simulink model "CN_filter"  (R2015b)
settings: Solver=VariableStepAuto  StartTime=0.0  StopTime=10.0  RelTol=1e-3
values from neighbouring files (symbols this model uses):
  FS = 0.2    [demo_DMC.m]
  TH = 1    [demo_DMC.m]
settings Model: Creator=mgreiff  LastModifiedBy=mgreiff

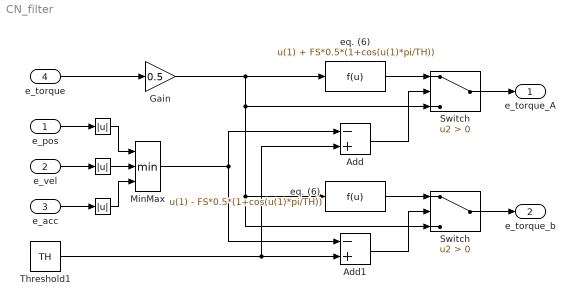
== system CN_filter ==
  e_pos : Inport
  "e_vel " : Inport  Port=2
  e_acc : Inport  Port=3
  e_torque : Inport  Port=4
  " " : Abs
  "  " : Abs
  "   " : Abs
  " Switch " : Switch  Criteria=u2 > Threshold
  " eq. (6) " : Fcn  Expr=u(1) + FS*0.5*(1+cos(u(1)*pi/TH))
  Add : Sum  Inputs=-+
  Add1 : Sum  Inputs=-+
  Gain : Gain  Gain=0.5
  MinMax : MinMax  Inputs=3
  Switch : Switch  Criteria=u2 > Threshold
  Threshold1 : Constant  Value=TH
  eq. (6) : Fcn  Expr=u(1) - FS*0.5*(1+cos(u(1)*pi/TH))
  e_torque_A : Outport
  e_torque_b : Outport  Port=2
  wires:
  Switch/1 -> e_torque_A/1
  " Switch "/1 -> e_torque_b/1
  e_torque/1 -> Gain/1
  Threshold1/1 -> Add/2, Add1/2
  Add/1 -> Switch/2
  Add1/1 -> " Switch "/2
  " eq. (6) "/1 -> Switch/1
  eq. (6)/1 -> " Switch "/1
  Gain/1 -> eq. (6)/1, " Switch "/3, Switch/3, " eq. (6) "/1
  MinMax/1 -> Add/1, Add1/1
  e_pos/1 -> " "/1
  "e_vel "/1 -> "   "/1
  e_acc/1 -> "  "/1
  " "/1 -> MinMax/1
  "  "/1 -> MinMax/3
  "   "/1 -> MinMax/2
